simulink model "IEEE9_16b_Rockefeller_uderen"  (R2020a)
settings: Solver=ode8  StartTime=0.0  StopTime=5  MaxStep=1e-4  RelTol=1e-3
undefined symbols (not defined in the file or in its folder): k
libraries: powerlib x33, powerlib_meascontrol x27, simulink_extras x24, dspsigops x6, sps_avr x3
(part 2 of 2)

== system IEEE9_16b_Rockefeller_uderen/192 MW ==
  note: 18kV 192 MVA
  192 MVA : powerlib/Machines/Synchronous Machine pu Standard  PresetModel=No  MechanicalLoad=Mechanical power Pm  ShowDetailedParameters=on  RotorType=Salient-pole  Units=per unit standard parameters  MeasurementBus=off  NominalParameters="[192e6  18000   60 ]"  Reactances1=[ 31 32 33 34 35 36 37 ]  Reactances2=[ 1.305, 0.296, 0.252, 0.474, 0.243, 0.18 ]  dAxisTimeConstants=Short-circuit  qAxisTimeConstants=Open-circuit  TimeConstants1=[]  TimeConstants2=[]  TimeConstants3=[]  TimeConstants4=[]  TimeConstants5=[ 1.01, 0.053, 0.1 ]  TimeConstants6=[]  TimeConstants7=[]  TimeConstants8=[]  StatorResistance=2.8544e-3  Mechanical="[20 0  32]"  PolePairs=32  InitialConditions=[0 -73.0594 0.600015 0.600015 0.600015 0.71576 -119.284 120.716 1.18255]  SetSaturation=off  Saturation=[0.6404,0.7127,0.8441,0.9214,0.9956,1.082,1.19,1.316,1.457;0.7,0.7698,0.8872,0.9466,0.9969,1.046,1.1,1.151,1.201]  LoadFlowParameters=[1 500000000 0 0 0]  TsPowergui=0  TsBlock=-1  IterativeModel=Trapezoidal non iterative  IterativeDiscreteModel=Trapezoidal non iterative  BusType=PV  Pref=0.6*192e6  Qref=0  Qmin=-Inf  Qmax=Inf  PLF=0  QLF=0
      settings: AttributesFormatString=\n\n
  Pref3 : Constant  Value=0.6
  Reg_M1 : Subsystem
  A : PMIOPort  Side=Right
  B : PMIOPort  Port=2  Side=Right
  C : PMIOPort  Port=3  Side=Right
  wires:
  Reg_M1/1(Pm) -> 192 MVA/1
  192 MVA/1 -> Reg_M1/1(m)
  Reg_M1/2(Vf) -> 192 MVA/2
  Pref3/1 -> Reg_M1/2(Pref)
  connections:
  192 MVA/RConn1 -- A/RConn1
  192 MVA/RConn3 -- C/RConn1
  192 MVA/RConn2 -- B/RConn1

== system IEEE9_16b_Rockefeller_uderen/247.5 MW ==
  note: 16.5kV 247.5 MVA
  247.5 MVA : powerlib/Machines/Synchronous Machine pu Standard  PresetModel=No  MechanicalLoad=Mechanical power Pm  ShowDetailedParameters=on  RotorType=Salient-pole  Units=per unit standard parameters  MeasurementBus=off  NominalParameters="[247.5e6  16500   60 ]"  Reactances1=[ 31 32 33 34 35 36 37 ]  Reactances2=[ 1.305, 0.296, 0.252, 0.474, 0.243, 0.18 ]  dAxisTimeConstants=Short-circuit  qAxisTimeConstants=Open-circuit  TimeConstants1=[]  TimeConstants2=[]  TimeConstants3=[]  TimeConstants4=[]  TimeConstants5=[ 1.01, 0.053, 0.1 ]  TimeConstants6=[]  TimeConstants7=[]  TimeConstants8=[]  StatorResistance=2.8544e-3  Mechanical=[20 0 32]  PolePairs=32  InitialConditions=[0 -76.6925 0.514814 0.514814 0.514814 -5.74321 -125.743 114.257 1.19383]  SetSaturation=off  Saturation=[0.6404,0.7127,0.8441,0.9214,0.9956,1.082,1.19,1.316,1.457;0.7,0.7698,0.8872,0.9466,0.9969,1.046,1.1,1.151,1.201]  LoadFlowParameters=[1 500000000 0 0 0]  TsPowergui=0  TsBlock=-1  IterativeModel=Trapezoidal non iterative  IterativeDiscreteModel=Trapezoidal non iterative  BusType=swing  Pref=5e+008  Qref=0  Qmin=-Inf  Qmax=Inf  PLF=0  QLF=0
      settings: AttributesFormatString=\n\n
  Pref3 : Constant  Value=0.51223
  Reg_M1 : Subsystem
  A : PMIOPort  Side=Right
  B : PMIOPort  Port=2  Side=Right
  C : PMIOPort  Port=3  Side=Right
  wires:
  Reg_M1/1(Pm) -> 247.5 MVA/1
  Reg_M1/2(Vf) -> 247.5 MVA/2
  Pref3/1 -> Reg_M1/2(Pref)
  247.5 MVA/1 -> Reg_M1/1(m)
  connections:
  A/RConn1 -- 247.5 MVA/RConn1
  247.5 MVA/RConn2 -- B/RConn1
  247.5 MVA/RConn3 -- C/RConn1

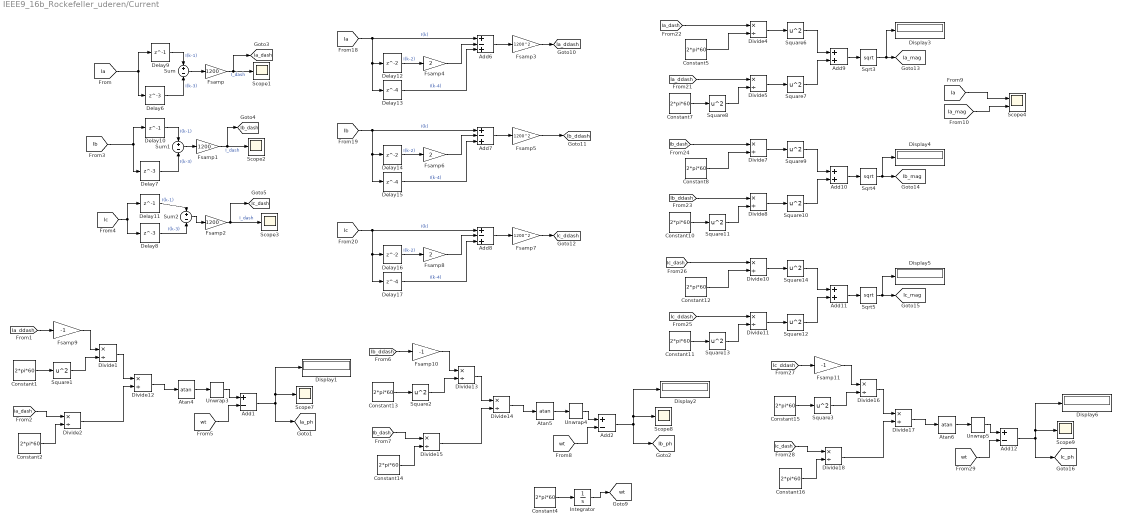
== system IEEE9_16b_Rockefeller_uderen/Current  ==
  Add1 : Sum  Inputs=+-
  Add10 : Sum
  Add11 : Sum
  Add12 : Sum  Inputs=+-
  Add2 : Sum  Inputs=+-
  Add6 : Sum  Inputs=+-+
  Add7 : Sum  Inputs=+-+
  Add8 : Sum  Inputs=+-+
  Add9 : Sum
  Atan4 : Trigonometry  Operator=atan
  Atan5 : Trigonometry  Operator=atan
  Atan6 : Trigonometry  Operator=atan
  Constant{1..2,4..5,7..8,10..16} (13 alike) : Constant  Value=2*pi*60
  Delay10 : Delay  DelayLength=1  SampleTime=1/1200
  Delay11 : Delay  DelayLength=1  SampleTime=1/1200
  Delay12 : Delay  SampleTime=1/1200
  Delay13 : Delay  DelayLength=4  SampleTime=1/1200
  Delay14 : Delay  SampleTime=1/1200
  Delay15 : Delay  DelayLength=4  SampleTime=1/1200
  Delay16 : Delay  SampleTime=1/1200
  Delay17 : Delay  DelayLength=4  SampleTime=1/1200
  Delay6 : Delay  DelayLength=3  SampleTime=1/1200
  Delay7 : Delay  DelayLength=3  SampleTime=1/1200
  Delay8 : Delay  DelayLength=3  SampleTime=1/1200
  Delay9 : Delay  DelayLength=1  SampleTime=1/1200
  Display{1..6} (6 alike) : Display
  Divide{1..2,4..5,7..8,10..18} (15 alike) : Product  Inputs=*/
  Fsamp : Gain  Gain=1200
  Fsamp1 : Gain  Gain=1200
  Fsamp10 : Gain  Gain=-1
  Fsamp11 : Gain  Gain=-1
  Fsamp2 : Gain  Gain=1200
  Fsamp3 : Gain  Gain=1200^2
  Fsamp4 : Gain  Gain=2
  Fsamp5 : Gain  Gain=1200^2
  Fsamp6 : Gain  Gain=2
  Fsamp7 : Gain  Gain=1200^2
  Fsamp8 : Gain  Gain=2
  Fsamp9 : Gain  Gain=-1
  Integrator : Integrator  WrappedStateUpperValue=2*pi  WrappedStateLowerValue=0
  Scope{1..3,7..9} (6 alike) : Scope
  Scope4 : Scope  NumInputPorts=2
  Sqrt3 : Sqrt  SaturateOnIntegerOverflow=on
  Sqrt4 : Sqrt  SaturateOnIntegerOverflow=on
  Sqrt5 : Sqrt  SaturateOnIntegerOverflow=on
  Square{1..3,6..14} (12 alike) : Math  Operator=square  SaturateOnIntegerOverflow=on
  Sum : Sum  Inputs=+-
  Sum1 : Sum  Inputs=+-
  Sum2 : Sum  Inputs=+-
  Unwrap3 : dspsigops/Unwrap  tol=-2*pi  InputProcessing=Columns as channels (frame based)  running=off
  Unwrap4 : dspsigops/Unwrap  tol=-2*pi  InputProcessing=Columns as channels (frame based)  running=off
  Unwrap5 : dspsigops/Unwrap  tol=-2*pi  InputProcessing=Columns as channels (frame based)  running=off
  tag scope: Ia_dash=global, Ia_ddash=global, Ia_mag=global, Ia_ph=global, Ib_dash=global, Ib_ddash=global, Ib_mag=global, Ib_ph=global, Ic_dash=global, Ic_ddash=global, Ic_mag=global, Ic_ph=global, wt=global
  wires:
  Delay6/1 -> Sum/2  "I(k-3)"
  [Ia] -> Delay6/1, Delay9/1
  Fsamp2/1 -> [Ic_dash], Scope3/1  "I_dash"
  Fsamp/1 -> [Ia_dash], Scope1/1  "I_dash"
  Sum1/1 -> Fsamp1/1
  Sum/1 -> Fsamp/1
  Constant4/1 -> Integrator/1
  Integrator/1 -> [wt]
  Delay9/1 -> Sum/1  "I(k-1)"
  Delay10/1 -> Sum1/1  "I(k-1)"
  [Ib] -> Delay7/1, Delay10/1
  Delay7/1 -> Sum1/2  "I(k-3)"
  Fsamp1/1 -> [Ib_dash], Scope2/1  "I_dash"
  Delay11/1 -> Sum2/1  "I(k-1)"
  [Ic] -> Delay8/1, Delay11/1
  Delay8/1 -> Sum2/2  "I(k-3)"
  Sum2/1 -> Fsamp2/1
  Delay12/1 -> Fsamp4/1  "I(k-2)"
  [Ia] -> Delay13/1, Delay12/1, Add6/1  "I(k)"
  Fsamp4/1 -> Add6/2
  Delay13/1 -> Add6/3  "I(k-4)"
  Add6/1 -> Fsamp3/1
  Fsamp3/1 -> [Ia_ddash]
  Fsamp5/1 -> [Ib_ddash]
  Add7/1 -> Fsamp5/1
  Delay15/1 -> Add7/3  "I(k-4)"
  Fsamp6/1 -> Add7/2
  [Ib] -> Add7/1, Delay14/1, Delay15/1  "I(k)"
  Delay14/1 -> Fsamp6/1  "I(k-2)"
  Delay16/1 -> Fsamp8/1  "I(k-2)"
  [Ic] -> Delay17/1, Delay16/1, Add8/1  "I(k)"
  Fsamp8/1 -> Add8/2
  Delay17/1 -> Add8/3  "I(k-4)"
  Add8/1 -> Fsamp7/1
  Fsamp7/1 -> [Ic_ddash]
  Constant5/1 -> Divide4/2
  Divide4/1 -> Square6/1
  [Ia_ddash] -> Divide5/1
  Divide5/1 -> Square7/1
  Constant7/1 -> Square8/1
  Square8/1 -> Divide5/2
  Square6/1 -> Add9/1
  Square7/1 -> Add9/2
  Add9/1 -> Sqrt3/1
  Sqrt3/1 -> Display3/1, [Ia_mag]
  Sqrt4/1 -> Display4/1, [Ib_mag]
  Add10/1 -> Sqrt4/1
  Square10/1 -> Add10/2
  Square9/1 -> Add10/1
  Square11/1 -> Divide8/2
  Constant10/1 -> Square11/1
  Divide8/1 -> Square10/1
  [Ib_ddash] -> Divide8/1
  Divide7/1 -> Square9/1
  Constant8/1 -> Divide7/2
  Constant12/1 -> Divide10/2
  Divide10/1 -> Square14/1
  [Ic_ddash] -> Divide11/1
  Divide11/1 -> Square12/1
  Constant11/1 -> Square13/1
  Square13/1 -> Divide11/2
  Square14/1 -> Add11/1
  Square12/1 -> Add11/2
  Add11/1 -> Sqrt5/1
  Sqrt5/1 -> Display5/1, [Ic_mag]
  [Ia_dash] -> Divide4/1
  [Ib_dash] -> Divide7/1
  [Ic_dash] -> Divide10/1
  [Ia_ddash] -> Fsamp9/1
  Constant1/1 -> Square1/1
  Fsamp9/1 -> Divide1/1
  Square1/1 -> Divide1/2
  [Ia_dash] -> Divide2/1
  Constant2/1 -> Divide2/2
  Divide1/1 -> Divide12/1
  Divide2/1 -> Divide12/2
  Divide12/1 -> Atan4/1
  Atan4/1 -> Unwrap3/1
  Unwrap3/1 -> Add1/1
  [wt] -> Add1/2
  Add1/1 -> Display1/1, Scope7/1, [Ia_ph]
  Add2/1 -> [Ib_ph], Scope8/1, Display2/1
  [wt] -> Add2/2
  Unwrap4/1 -> Add2/1
  Atan5/1 -> Unwrap4/1
  Divide14/1 -> Atan5/1
  Divide15/1 -> Divide14/2
  Divide13/1 -> Divide14/1
  Constant14/1 -> Divide15/2
  [Ib_dash] -> Divide15/1
  Square2/1 -> Divide13/2
  Fsamp10/1 -> Divide13/1
  Constant13/1 -> Square2/1
  [Ib_ddash] -> Fsamp10/1
  [Ic_ddash] -> Fsamp11/1
  Constant15/1 -> Square3/1
  Fsamp11/1 -> Divide16/1
  Square3/1 -> Divide16/2
  [Ic_dash] -> Divide18/1
  Constant16/1 -> Divide18/2
  Divide16/1 -> Divide17/1
  Divide18/1 -> Divide17/2
  Divide17/1 -> Atan6/1
  Atan6/1 -> Unwrap5/1
  Unwrap5/1 -> Add12/1
  [wt] -> Add12/2
  Add12/1 -> Display6/1, Scope9/1, [Ic_ph]
  [Ia] -> Scope4/1
  [Ia_mag] -> Scope4/2

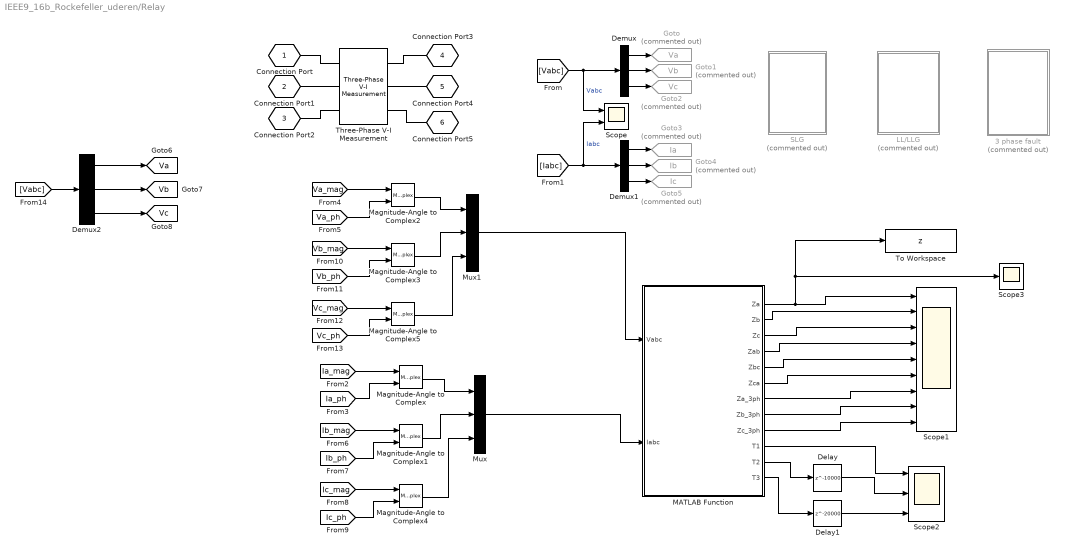
== system IEEE9_16b_Rockefeller_uderen/Relay ==
  3 phase fault : Subsystem  Commented=on
  Delay : Delay  DelayLength=10000  SampleTime=50e-6
  Delay1 : Delay  DelayLength=20000  SampleTime=50e-6
  Demux : Demux  Outputs=3
  Demux1 : Demux  Outputs=3
  Demux2 : Demux  Outputs=3
  Goto : Goto  Commented=on  GotoTag=Va  TagVisibility=global
  Goto1 : Goto  Commented=on  GotoTag=Vb  TagVisibility=global
  Goto2 : Goto  Commented=on  GotoTag=Vc  TagVisibility=global
  Goto3 : Goto  Commented=on  GotoTag=Ia  TagVisibility=global
  Goto4 : Goto  Commented=on  GotoTag=Ib  TagVisibility=global
  Goto5 : Goto  Commented=on  GotoTag=Ic  TagVisibility=global
  LL/LLG : Subsystem  Commented=on
  MATLAB Function : MATLAB Function  TreatAsAtomicUnit=on
  Magnitude-Angle to Complex{,1..5} (6 alike) : MagnitudeAngleToComplex
  Mux : Mux  Inputs=3
  Mux1 : Mux  Inputs=3
  SLG : Subsystem  Commented=on
  Scope : Scope  NumInputPorts=2
  Scope1 : Scope  NumInputPorts=9
  Scope2 : Scope  NumInputPorts=3
  Scope3 : Scope
  Three-Phase V-I Measurement : powerlib/Measurements/Three-Phase V-I Measurement  VoltageMeasurement=phase-to-ground  SetLabelV=on  LabelV=Vabc  Vpu=off  VpuLL=off  CurrentMeasurement=yes  SetLabelI=on  LabelI=Iabc  Ipu=off  Pbase=100e6  Vbase=500e3  OutputType=Complex  PhasorSimulation=off  PSBequivalent=0
  To Workspace : ToWorkspace  VariableName=z  SampleTime=-1
  Connection Port : PMIOPort  Tag=PMCPort  Side=Left
  Connection Port1 : PMIOPort  Tag=PMCPort  Port=2  Side=Left
  Connection Port2 : PMIOPort  Tag=PMCPort  Port=3  Side=Left
  Connection Port3 : PMIOPort  Tag=PMCPort  Port=4  Side=Right
  Connection Port4 : PMIOPort  Tag=PMCPort  Port=5  Side=Right
  Connection Port5 : PMIOPort  Tag=PMCPort  Port=6  Side=Right
  tag scope: Va=global, Vb=global, Vc=global
  wires:
  Demux1/3 -> Goto5/1
  Demux1/1 -> Goto3/1
  Demux/3 -> Goto2/1
  Demux/1 -> Goto/1
  Demux/2 -> Goto1/1
  [Iabc] -> Scope/2, Demux1/1  "Iabc"
  [Vabc] -> Scope/1, Demux/1  "Vabc"
  Demux1/2 -> Goto4/1
  MATLAB Function/1(Za) -> Scope3/1, To Workspace/1, Scope1/1
  MATLAB Function/2(Zb) -> Scope1/2
  MATLAB Function/3(Zc) -> Scope1/3
  MATLAB Function/4(Zab) -> Scope1/4
  MATLAB Function/5(Zbc) -> Scope1/5
  MATLAB Function/6(Zca) -> Scope1/6
  MATLAB Function/10(T1) -> Scope2/1
  Mux/1 -> MATLAB Function/2(Iabc)
  MATLAB Function/11(T2) -> Delay/1
  MATLAB Function/12(T3) -> Delay1/1
  Delay/1 -> Scope2/2
  Delay1/1 -> Scope2/3
  MATLAB Function/7(Za_3ph) -> Scope1/7
  MATLAB Function/8(Zb_3ph) -> Scope1/8
  MATLAB Function/9(Zc_3ph) -> Scope1/9
  [Ia_mag] -> Magnitude-Angle to Complex/1
  [Ia_ph] -> Magnitude-Angle to Complex/2
  [Ib_ph] -> Magnitude-Angle to Complex1/2
  [Ib_mag] -> Magnitude-Angle to Complex1/1
  [Ic_mag] -> Magnitude-Angle to Complex4/1
  [Ic_ph] -> Magnitude-Angle to Complex4/2
  Magnitude-Angle to Complex/1 -> Mux/1
  Magnitude-Angle to Complex1/1 -> Mux/2
  Magnitude-Angle to Complex4/1 -> Mux/3
  Magnitude-Angle to Complex5/1 -> Mux1/3
  Magnitude-Angle to Complex3/1 -> Mux1/2
  Magnitude-Angle to Complex2/1 -> Mux1/1
  [Vc_ph] -> Magnitude-Angle to Complex5/2
  [Vc_mag] -> Magnitude-Angle to Complex5/1
  [Vb_mag] -> Magnitude-Angle to Complex3/1
  [Vb_ph] -> Magnitude-Angle to Complex3/2
  [Va_ph] -> Magnitude-Angle to Complex2/2
  [Va_mag] -> Magnitude-Angle to Complex2/1
  Mux1/1 -> MATLAB Function/1(Vabc)
  [Vabc] -> Demux2/1
  Demux2/1 -> [Va]
  Demux2/2 -> [Vb]
  Demux2/3 -> [Vc]
  connections:
  Connection Port/RConn1 -- Three-Phase V-I Measurement/LConn1
  Connection Port1/RConn1 -- Three-Phase V-I Measurement/LConn2
  Connection Port2/RConn1 -- Three-Phase V-I Measurement/LConn3
  Connection Port3/RConn1 -- Three-Phase V-I Measurement/RConn1
  Connection Port4/RConn1 -- Three-Phase V-I Measurement/RConn2
  Connection Port5/RConn1 -- Three-Phase V-I Measurement/RConn3

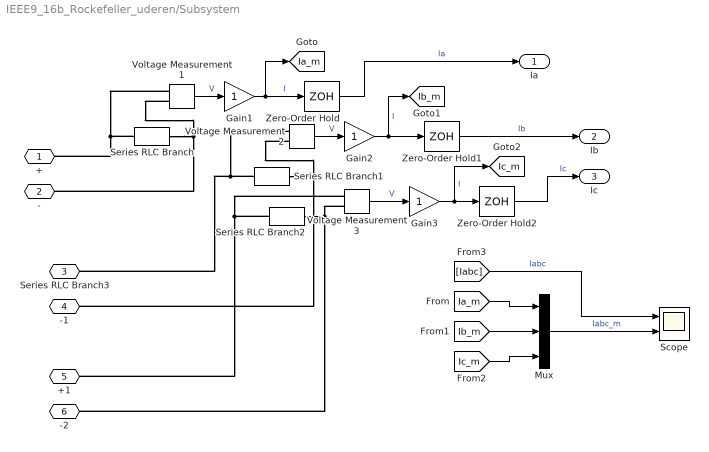
== system IEEE9_16b_Rockefeller_uderen/Subsystem ==
  Gain1 : Gain
  Gain2 : Gain
  Gain3 : Gain
  Mux : Mux  Inputs=3
  Scope : Scope  NumInputPorts=2
  Series RLC Branch : powerlib/Elements/Series RLC Branch  LConnTagsString=__new0  RConnTagsString=__new0  BranchType=RL  Resistance=0.11727  Inductance=2.634e-3  SetiL0=off  InitialCurrent=0  Capacitance=1e-6  Setx0=off  InitialVoltage=0  Measurements=None
  Series RLC Branch1 : powerlib/Elements/Series RLC Branch  LConnTagsString=__new0  RConnTagsString=__new0  BranchType=RL  Resistance=0.11727  Inductance=2.634e-3  SetiL0=off  InitialCurrent=0  Capacitance=1e-6  Setx0=off  InitialVoltage=0  Measurements=None
  Series RLC Branch2 : powerlib/Elements/Series RLC Branch  LConnTagsString=__new0  RConnTagsString=__new0  BranchType=RL  Resistance=0.11727  Inductance=2.634e-3  SetiL0=off  InitialCurrent=0  Capacitance=1e-6  Setx0=off  InitialVoltage=0  Measurements=None
  Voltage Measurement1 : powerlib/Measurements/Voltage Measurement  PhasorSimulation=off  OutputType=Complex  PSBequivalent=0
  Voltage Measurement2 : powerlib/Measurements/Voltage Measurement  PhasorSimulation=off  OutputType=Complex  PSBequivalent=0
  Voltage Measurement3 : powerlib/Measurements/Voltage Measurement  PhasorSimulation=off  OutputType=Complex  PSBequivalent=0
  Zero-Order Hold : ZeroOrderHold  SampleTime=1/1200
  Zero-Order Hold1 : ZeroOrderHold  SampleTime=1/1200
  Zero-Order Hold2 : ZeroOrderHold  SampleTime=1/1200
  + : PMIOPort  Side=Left
  - : PMIOPort  Port=2  Side=Left
  Series RLC Branch3 : PMIOPort  Port=3  Side=Left
  -1 : PMIOPort  Port=4  Side=Left
  +1 : PMIOPort  Port=5  Side=Left
  -2 : PMIOPort  Port=6  Side=Left
  Ia : Outport
  Ib : Outport  Port=2
  Ic : Outport  Port=3
  tag scope: Ia_m=global, Ib_m=global, Ic_m=global
  wires:
  Voltage Measurement1/1 -> Gain1/1  "V"
  Gain1/1 -> [Ia_m], Zero-Order Hold/1  "I"
  Voltage Measurement2/1 -> Gain2/1  "V"
  Gain2/1 -> [Ib_m], Zero-Order Hold1/1  "I"
  Zero-Order Hold1/1 -> Ib/1  "Ib"
  Voltage Measurement3/1 -> Gain3/1  "V"
  Gain3/1 -> [Ic_m], Zero-Order Hold2/1  "I"
  Zero-Order Hold/1 -> Ia/1  "Ia"
  Zero-Order Hold2/1 -> Ic/1  "Ic"
  [Ib_m] -> Mux/2
  [Ic_m] -> Mux/3
  [Ia_m] -> Mux/1
  Mux/1 -> Scope/2  "Iabc_m"
  [Iabc] -> Scope/1  "Iabc"
  connections:
  Series RLC Branch2/LConn1 -- +1/RConn1 -- Voltage Measurement3/LConn1
  Series RLC Branch/LConn1 -- +/RConn1 -- Voltage Measurement1/LConn1
  Series RLC Branch2/RConn1 -- -2/RConn1 -- Voltage Measurement3/LConn2
  Series RLC Branch1/RConn1 -- -1/RConn1 -- Voltage Measurement2/LConn2
  Voltage Measurement2/LConn1 -- Series RLC Branch3/RConn1 -- Series RLC Branch1/LConn1
  Series RLC Branch/RConn1 -- -/RConn1 -- Voltage Measurement1/LConn2

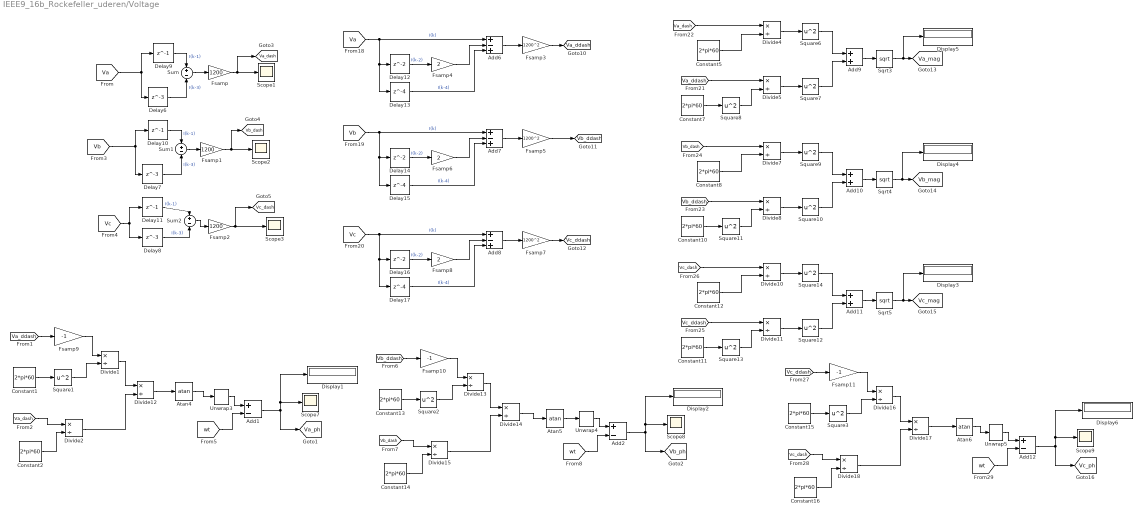
== system IEEE9_16b_Rockefeller_uderen/Voltage ==
  Add1 : Sum  Inputs=+-
  Add10 : Sum
  Add11 : Sum
  Add12 : Sum  Inputs=+-
  Add2 : Sum  Inputs=+-
  Add6 : Sum  Inputs=+-+
  Add7 : Sum  Inputs=+-+
  Add8 : Sum  Inputs=+-+
  Add9 : Sum
  Atan4 : Trigonometry  Operator=atan
  Atan5 : Trigonometry  Operator=atan
  Atan6 : Trigonometry  Operator=atan
  Constant{1..2,5,7..8,10..16} (12 alike) : Constant  Value=2*pi*60
  Delay10 : Delay  DelayLength=1  SampleTime=1/1200
  Delay11 : Delay  DelayLength=1  SampleTime=1/1200
  Delay12 : Delay  SampleTime=1/1200
  Delay13 : Delay  DelayLength=4  SampleTime=1/1200
  Delay14 : Delay  SampleTime=1/1200
  Delay15 : Delay  DelayLength=4  SampleTime=1/1200
  Delay16 : Delay  SampleTime=1/1200
  Delay17 : Delay  DelayLength=4  SampleTime=1/1200
  Delay6 : Delay  DelayLength=3  SampleTime=1/1200
  Delay7 : Delay  DelayLength=3  SampleTime=1/1200
  Delay8 : Delay  DelayLength=3  SampleTime=1/1200
  Delay9 : Delay  DelayLength=1  SampleTime=1/1200
  Display{1..6} (6 alike) : Display
  Divide{1..2,4..5,7..8,10..18} (15 alike) : Product  Inputs=*/
  Fsamp : Gain  Gain=1200
  Fsamp1 : Gain  Gain=1200
  Fsamp10 : Gain  Gain=-1
  Fsamp11 : Gain  Gain=-1
  Fsamp2 : Gain  Gain=1200
  Fsamp3 : Gain  Gain=1200^2
  Fsamp4 : Gain  Gain=2
  Fsamp5 : Gain  Gain=1200^2
  Fsamp6 : Gain  Gain=2
  Fsamp7 : Gain  Gain=1200^2
  Fsamp8 : Gain  Gain=2
  Fsamp9 : Gain  Gain=-1
  Scope{1..3,7..9} (6 alike) : Scope
  Sqrt3 : Sqrt  SaturateOnIntegerOverflow=on
  Sqrt4 : Sqrt  SaturateOnIntegerOverflow=on
  Sqrt5 : Sqrt  SaturateOnIntegerOverflow=on
  Square{1..3,6..14} (12 alike) : Math  Operator=square  SaturateOnIntegerOverflow=on
  Sum : Sum  Inputs=+-
  Sum1 : Sum  Inputs=+-
  Sum2 : Sum  Inputs=+-
  Unwrap3 : dspsigops/Unwrap  tol=-2*pi  InputProcessing=Columns as channels (frame based)  running=off
  Unwrap4 : dspsigops/Unwrap  tol=-2*pi  InputProcessing=Columns as channels (frame based)  running=off
  Unwrap5 : dspsigops/Unwrap  tol=-2*pi  InputProcessing=Columns as channels (frame based)  running=off
  tag scope: Va_dash=global, Va_ddash=global, Va_mag=global, Va_ph=global, Vb_dash=global, Vb_ddash=global, Vb_mag=global, Vb_ph=global, Vc_dash=global, Vc_ddash=global, Vc_mag=global, Vc_ph=global
  wires:
  Add12/1 -> [Vc_ph], Scope9/1, Display6/1
  [wt] -> Add12/2
  Unwrap5/1 -> Add12/1
  Atan6/1 -> Unwrap5/1
  Divide17/1 -> Atan6/1
  Divide18/1 -> Divide17/2
  Divide16/1 -> Divide17/1
  Constant16/1 -> Divide18/2
  [Vc_dash] -> Divide18/1
  Square3/1 -> Divide16/2
  Fsamp11/1 -> Divide16/1
  Constant15/1 -> Square3/1
  [Vc_ddash] -> Fsamp11/1
  [Vb_ddash] -> Fsamp10/1
  Constant13/1 -> Square2/1
  Fsamp10/1 -> Divide13/1
  Square2/1 -> Divide13/2
  [Vb_dash] -> Divide15/1
  Constant14/1 -> Divide15/2
  Divide13/1 -> Divide14/1
  Divide15/1 -> Divide14/2
  Divide14/1 -> Atan5/1
  Atan5/1 -> Unwrap4/1
  Unwrap4/1 -> Add2/1
  [wt] -> Add2/2
  Add2/1 -> Display2/1, Scope8/1, [Vb_ph]
  Add1/1 -> [Va_ph], Scope7/1, Display1/1
  [wt] -> Add1/2
  Unwrap3/1 -> Add1/1
  Atan4/1 -> Unwrap3/1
  Divide12/1 -> Atan4/1
  Divide2/1 -> Divide12/2
  Divide1/1 -> Divide12/1
  Constant2/1 -> Divide2/2
  [Va_dash] -> Divide2/1
  Square1/1 -> Divide1/2
  Fsamp9/1 -> Divide1/1
  Constant1/1 -> Square1/1
  [Va_ddash] -> Fsamp9/1
  [Vc_dash] -> Divide10/1
  [Vb_dash] -> Divide7/1
  [Va_dash] -> Divide4/1
  Sqrt5/1 -> Display3/1, [Vc_mag]
  Add11/1 -> Sqrt5/1
  Square12/1 -> Add11/2
  Square14/1 -> Add11/1
  Square13/1 -> Divide11/2
  Constant11/1 -> Square13/1
  Divide11/1 -> Square12/1
  [Vc_ddash] -> Divide11/1
  Divide10/1 -> Square14/1
  Constant12/1 -> Divide10/2
  Constant8/1 -> Divide7/2
  Divide7/1 -> Square9/1
  [Vb_ddash] -> Divide8/1
  Divide8/1 -> Square10/1
  Constant10/1 -> Square11/1
  Square11/1 -> Divide8/2
  Square9/1 -> Add10/1
  Square10/1 -> Add10/2
  Add10/1 -> Sqrt4/1
  Sqrt4/1 -> Display4/1, [Vb_mag]
  Sqrt3/1 -> Display5/1, [Va_mag]
  Add9/1 -> Sqrt3/1
  Square7/1 -> Add9/2
  Square6/1 -> Add9/1
  Square8/1 -> Divide5/2
  Constant7/1 -> Square8/1
  Divide5/1 -> Square7/1
  [Va_ddash] -> Divide5/1
  Divide4/1 -> Square6/1
  Constant5/1 -> Divide4/2
  Fsamp7/1 -> [Vc_ddash]
  Add8/1 -> Fsamp7/1
  Delay17/1 -> Add8/3  "I(k-4)"
  Fsamp8/1 -> Add8/2
  [Vc] -> Add8/1, Delay16/1, Delay17/1  "I(k)"
  Delay16/1 -> Fsamp8/1  "I(k-2)"
  Delay14/1 -> Fsamp6/1  "I(k-2)"
  [Vb] -> Delay15/1, Delay14/1, Add7/1  "I(k)"
  Fsamp6/1 -> Add7/2
  Delay15/1 -> Add7/3  "I(k-4)"
  Add7/1 -> Fsamp5/1
  Fsamp5/1 -> [Vb_ddash]
  Fsamp3/1 -> [Va_ddash]
  Add6/1 -> Fsamp3/1
  Delay13/1 -> Add6/3  "I(k-4)"
  Fsamp4/1 -> Add6/2
  [Va] -> Add6/1, Delay12/1, Delay13/1  "I(k)"
  Delay12/1 -> Fsamp4/1  "I(k-2)"
  Sum2/1 -> Fsamp2/1
  Delay8/1 -> Sum2/2  "I(k-3)"
  [Vc] -> Delay11/1, Delay8/1
  Delay11/1 -> Sum2/1  "I(k-1)"
  Fsamp1/1 -> Scope2/1, [Vb_dash]
  Delay7/1 -> Sum1/2  "I(k-3)"
  [Vb] -> Delay10/1, Delay7/1
  Delay10/1 -> Sum1/1  "I(k-1)"
  Delay9/1 -> Sum/1  "I(k-1)"
  Sum/1 -> Fsamp/1
  Sum1/1 -> Fsamp1/1
  Fsamp/1 -> Scope1/1, [Va_dash]
  Fsamp2/1 -> Scope3/1, [Vc_dash]
  [Va] -> Delay9/1, Delay6/1
  Delay6/1 -> Sum/2  "I(k-3)"

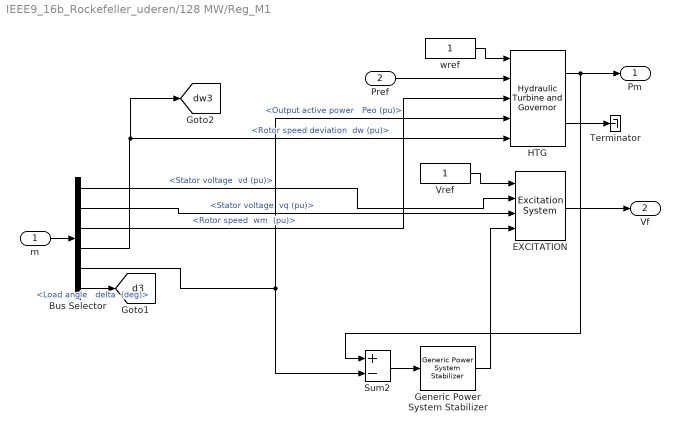
== system IEEE9_16b_Rockefeller_uderen/128 MW/Reg_M1 ==
  m : Inport
  Pref : Inport  Port=2
  Bus Selector : BusSelector  OutputSignals="dq0 components.Stator voltage  vd (pu),dq0 components.Stator voltage  vq (pu),Mechanical.Rotor speed  wm  (pu),Mechanical.Rotor speed deviation  dw (pu),Output active power   Peo (pu),Load angle   delta  (deg)"
  EXCITATION : sps_avr/Excitation System  tr=20e-3  reg=[ 200, 0.001 ]  exc=[ 1, 0 ]  tgr=[ 0, 0 ]  damp=[ 0.001, 0.1 ]  sat=[ 0, 0 ]  lim="[ 0,  7, 0 ]"  v0=[1 1.1034]
      settings: SourceProductBaseCode=PS
  Generic Power System Stabilizer : powerlib/Machines/Generic Power System Stabilizer  Tsensor=15e-3  K=2.5  Twashout=1  Tleadlag1="[0.06  1]"  Tleadlag2="[0  0]"  VSlimits=[-0.15 0.15]  Vinit=0  Plot_On=off  MagdB_On=on  FreqRange=logspace(-2,2,500)
      settings: SourceProductBaseCode=PS
  HTG : powerlib/Machines/Hydraulic Turbine and Governor  sm="[ 10/3  0.07 ]"  gate="[  0.01  0.97518  -0.1  0.1 ]"  reg="[  0.05  1.163  0.105  0  0.01  ]"  hyd="[  0  2.67  ]"  dref=0  po=0.60104
      settings: SourceProductBaseCode=PS
  Sum2 : Sum  Inputs=+-  InputSameDT=on  SaturateOnIntegerOverflow=on  OutDataTypeStr=Inherit: Same as first input
  Terminator : Terminator
  Vref : Constant
  wref : Constant
  Pm : Outport  InitialOutput=0
  Vf : Outport  Port=2  InitialOutput=0
  tag scope: d3=global, dw3=global
  wires:
  HTG/2 -> Terminator/1
  Vref/1 -> EXCITATION/1
  m/1 -> Bus Selector/1
  Bus Selector/4 -> [dw3], HTG/5  "<Rotor speed deviation  dw (pu)>"
  Bus Selector/5 -> HTG/4, Sum2/2  "<Output active power   Peo (pu)>"
  Bus Selector/3 -> HTG/3  "<Rotor speed  wm  (pu)>"
  Pref/1 -> HTG/2
  wref/1 -> HTG/1
  HTG/1 -> Pm/1, Sum2/1
  Bus Selector/2 -> EXCITATION/3  "<Stator voltage  vq (pu)>"
  EXCITATION/1 -> Vf/1
  Bus Selector/1 -> EXCITATION/2  "<Stator voltage  vd (pu)>"
  Generic Power System Stabilizer/1 -> EXCITATION/4
  Sum2/1 -> Generic Power System Stabilizer/1
  Bus Selector/6 -> [d3]  "<Load angle   delta  (deg)>"

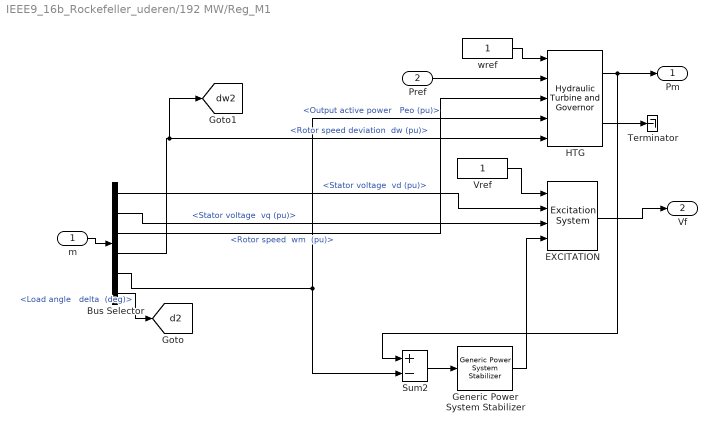
== system IEEE9_16b_Rockefeller_uderen/192 MW/Reg_M1 ==
  m : Inport
  Pref : Inport  Port=2
  Bus Selector : BusSelector  OutputSignals="dq0 components.Stator voltage  vd (pu),dq0 components.Stator voltage  vq (pu),Mechanical.Rotor speed  wm  (pu),Mechanical.Rotor speed deviation  dw (pu),Output active power   Peo (pu),Load angle   delta  (deg)"
  EXCITATION : sps_avr/Excitation System  tr=20e-3  reg=[ 200, 0.001 ]  exc=[ 1, 0 ]  tgr=[ 0, 0 ]  damp=[ 0.001, 0.1 ]  sat=[ 0, 0 ]  lim="[ 0,  7, 0 ]"  v0=[1 1.1826]
      settings: SourceProductBaseCode=PS
  Generic Power System Stabilizer : powerlib/Machines/Generic Power System Stabilizer  Tsensor=15e-3  K=2.5  Twashout=1  Tleadlag1="[0.06  1]"  Tleadlag2="[0  0]"  VSlimits=[-0.15 0.15]  Vinit=0  Plot_On=off  MagdB_On=on  FreqRange=logspace(-2,2,500)
      settings: SourceProductBaseCode=PS
  HTG : powerlib/Machines/Hydraulic Turbine and Governor  sm="[ 10/3  0.07 ]"  gate="[  0.01  0.97518  -0.1  0.1 ]"  reg="[  0.05  1.163  0.105  0  0.01  ]"  hyd="[  0  2.67  ]"  dref=0  po=0.60103
      settings: SourceProductBaseCode=PS
  Sum2 : Sum  Inputs=+-  InputSameDT=on  SaturateOnIntegerOverflow=on  OutDataTypeStr=Inherit: Same as first input
  Terminator : Terminator
  Vref : Constant
  wref : Constant
  Pm : Outport  InitialOutput=0
  Vf : Outport  Port=2  InitialOutput=0
  tag scope: d2=global, dw2=global
  wires:
  HTG/2 -> Terminator/1
  Vref/1 -> EXCITATION/1
  m/1 -> Bus Selector/1
  Bus Selector/4 -> [dw2], HTG/5  "<Rotor speed deviation  dw (pu)>"
  Bus Selector/5 -> HTG/4, Sum2/2  "<Output active power   Peo (pu)>"
  Bus Selector/3 -> HTG/3  "<Rotor speed  wm  (pu)>"
  Pref/1 -> HTG/2
  wref/1 -> HTG/1
  HTG/1 -> Pm/1, Sum2/1
  Bus Selector/2 -> EXCITATION/3  "<Stator voltage  vq (pu)>"
  EXCITATION/1 -> Vf/1
  Bus Selector/1 -> EXCITATION/2  "<Stator voltage  vd (pu)>"
  Generic Power System Stabilizer/1 -> EXCITATION/4
  Sum2/1 -> Generic Power System Stabilizer/1
  Bus Selector/6 -> [d2]  "<Load angle   delta  (deg)>"

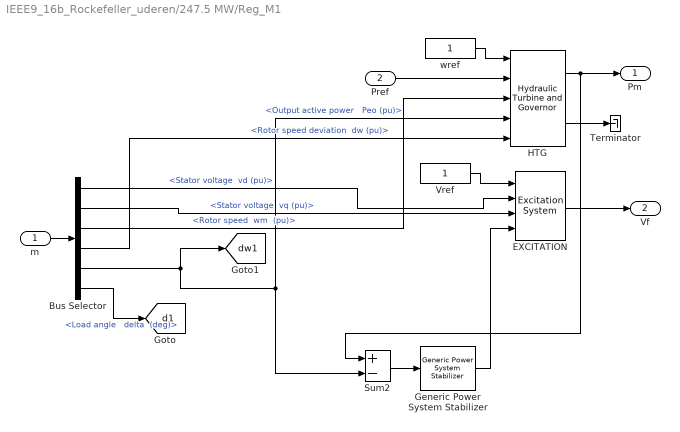
== system IEEE9_16b_Rockefeller_uderen/247.5 MW/Reg_M1 ==
  m : Inport
  Pref : Inport  Port=2
  Bus Selector : BusSelector  OutputSignals="dq0 components.Stator voltage  vd (pu),dq0 components.Stator voltage  vq (pu),Mechanical.Rotor speed  wm  (pu),Mechanical.Rotor speed deviation  dw (pu),Output active power   Peo (pu),Load angle   delta  (deg)"
  EXCITATION : sps_avr/Excitation System  tr=20e-3  reg=[ 200, 0.001 ]  exc=[ 1, 0 ]  tgr=[ 0, 0 ]  damp=[ 0.001, 0.1 ]  sat=[ 0, 0 ]  lim="[ 0,  7, 0 ]"  v0=[1 1.1938]
      settings: SourceProductBaseCode=PS
  Generic Power System Stabilizer : powerlib/Machines/Generic Power System Stabilizer  Tsensor=15e-3  K=2.5  Twashout=1  Tleadlag1="[0.06  1]"  Tleadlag2="[0  0]"  VSlimits=[-0.15 0.15]  Vinit=0  Plot_On=off  MagdB_On=on  FreqRange=logspace(-2,2,500)
      settings: SourceProductBaseCode=PS
  HTG : powerlib/Machines/Hydraulic Turbine and Governor  sm="[ 10/3  0.07 ]"  gate="[  0.01  0.97518  -0.1  0.1 ]"  reg="[  0.05  1.163  0.105  0  0.01  ]"  hyd="[  0  2.67  ]"  dref=0  po=0.51299
      settings: SourceProductBaseCode=PS
  Sum2 : Sum  Inputs=+-  InputSameDT=on  SaturateOnIntegerOverflow=on  OutDataTypeStr=Inherit: Same as first input
  Terminator : Terminator
  Vref : Constant
  wref : Constant
  Pm : Outport  InitialOutput=0
  Vf : Outport  Port=2  InitialOutput=0
  tag scope: d1=global, dw1=global
  wires:
  HTG/2 -> Terminator/1
  Vref/1 -> EXCITATION/1
  m/1 -> Bus Selector/1
  Bus Selector/4 -> HTG/5  "<Rotor speed deviation  dw (pu)>"
  Bus Selector/5 -> [dw1], HTG/4, Sum2/2  "<Output active power   Peo (pu)>"
  Bus Selector/3 -> HTG/3  "<Rotor speed  wm  (pu)>"
  Pref/1 -> HTG/2
  wref/1 -> HTG/1
  HTG/1 -> Pm/1, Sum2/1
  Bus Selector/2 -> EXCITATION/3  "<Stator voltage  vq (pu)>"
  EXCITATION/1 -> Vf/1
  Bus Selector/1 -> EXCITATION/2  "<Stator voltage  vd (pu)>"
  Generic Power System Stabilizer/1 -> EXCITATION/4
  Sum2/1 -> Generic Power System Stabilizer/1
  Bus Selector/6 -> [d1]  "<Load angle   delta  (deg)>"

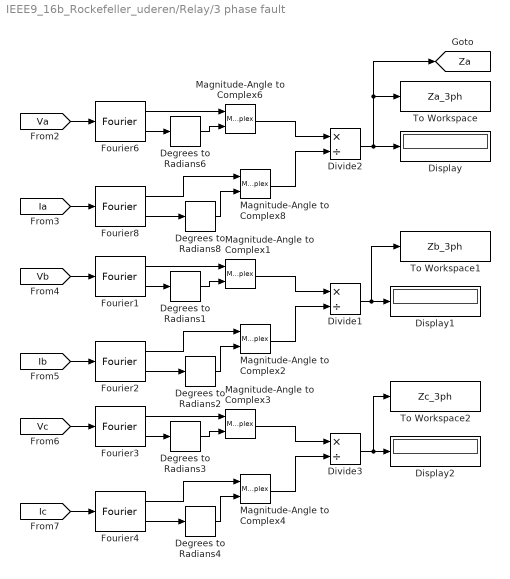
== system IEEE9_16b_Rockefeller_uderen/Relay/3 phase fault ==
  Degrees to Radians{1..4,6,8} (6 alike) : simulink_extras/Transformations/Degrees to Radians
  Display : Display
  Display1 : Display
  Display2 : Display
  Divide1 : Product  Inputs=*/
  Divide2 : Product  Inputs=*/
  Divide3 : Product  Inputs=*/
  Fourier{1..4,6,8} (6 alike) : powerlib_meascontrol/Measurements/Fourier  Freq=60  n=1  InInit=[0, 0]  Ts=0
  Magnitude-Angle to Complex{1..4,6,8} (6 alike) : MagnitudeAngleToComplex
  To Workspace : ToWorkspace  VariableName=Za_3ph  SaveFormat=Timeseries  SampleTime=-1
  To Workspace1 : ToWorkspace  VariableName=Zb_3ph  SaveFormat=Timeseries  SampleTime=-1
  To Workspace2 : ToWorkspace  VariableName=Zc_3ph  SaveFormat=Timeseries  SampleTime=-1
  tag scope: Za=global
  wires:
  Divide1/1 -> To Workspace1/1, Display1/1
  [Ia] -> Fourier8/1
  [Ib] -> Fourier2/1
  Degrees to Radians4/1 -> Magnitude-Angle to Complex4/2
  Magnitude-Angle to Complex3/1 -> Divide3/1
  Fourier4/2 -> Degrees to Radians4/1
  Degrees to Radians8/1 -> Magnitude-Angle to Complex8/2
  Fourier6/2 -> Degrees to Radians6/1
  Magnitude-Angle to Complex6/1 -> Divide2/1
  Magnitude-Angle to Complex8/1 -> Divide2/2
  Degrees to Radians2/1 -> Magnitude-Angle to Complex2/2
  Fourier8/2 -> Degrees to Radians8/1
  [Va] -> Fourier6/1
  Divide3/1 -> To Workspace2/1, Display2/1
  Fourier3/1 -> Magnitude-Angle to Complex3/1
  Degrees to Radians6/1 -> Magnitude-Angle to Complex6/2
  Divide2/1 -> [Za], To Workspace/1, Display/1
  Fourier6/1 -> Magnitude-Angle to Complex6/1
  Fourier8/1 -> Magnitude-Angle to Complex8/1
  Fourier2/2 -> Degrees to Radians2/1
  Fourier3/2 -> Degrees to Radians3/1
  Degrees to Radians1/1 -> Magnitude-Angle to Complex1/2
  [Vc] -> Fourier3/1
  Magnitude-Angle to Complex4/1 -> Divide3/2
  Fourier4/1 -> Magnitude-Angle to Complex4/1
  Fourier1/1 -> Magnitude-Angle to Complex1/1
  Degrees to Radians3/1 -> Magnitude-Angle to Complex3/2
  [Ic] -> Fourier4/1
  Magnitude-Angle to Complex2/1 -> Divide1/2
  Magnitude-Angle to Complex1/1 -> Divide1/1
  Fourier1/2 -> Degrees to Radians1/1
  [Vb] -> Fourier1/1
  Fourier2/1 -> Magnitude-Angle to Complex2/1

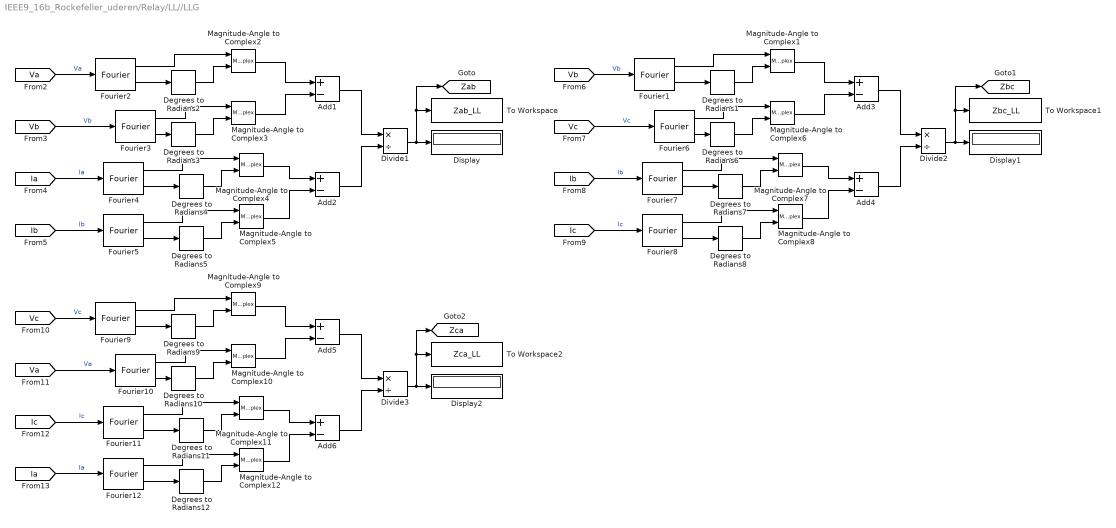
== system IEEE9_16b_Rockefeller_uderen/Relay/LL//LLG ==
  Add{1..6} (6 alike) : Sum  Inputs=+-
  Degrees to Radians{1..12} (12 alike) : simulink_extras/Transformations/Degrees to Radians
  Display : Display
  Display1 : Display
  Display2 : Display
  Divide1 : Product  Inputs=*/
  Divide2 : Product  Inputs=*/
  Divide3 : Product  Inputs=*/
  Fourier{1..12} (12 alike) : powerlib_meascontrol/Measurements/Fourier  Freq=60  n=1  InInit=[0, 0]  Ts=0
  Magnitude-Angle to Complex{1..12} (12 alike) : MagnitudeAngleToComplex
  To Workspace : ToWorkspace  VariableName=Zab_LL  SaveFormat=Timeseries  SampleTime=-1
  To Workspace1 : ToWorkspace  VariableName=Zbc_LL  SaveFormat=Timeseries  SampleTime=-1
  To Workspace2 : ToWorkspace  VariableName=Zca_LL  SaveFormat=Timeseries  SampleTime=-1
  tag scope: Zab=global, Zbc=global, Zca=global
  wires:
  Fourier12/2 -> Degrees to Radians12/1
  [Vc] -> Fourier9/1  "Vc"
  [Vc] -> Fourier6/1  "Vc"
  Magnitude-Angle to Complex11/1 -> Add6/1
  Fourier2/2 -> Degrees to Radians2/1
  Degrees to Radians8/1 -> Magnitude-Angle to Complex8/2
  Fourier10/1 -> Magnitude-Angle to Complex10/1
  Magnitude-Angle to Complex5/1 -> Add2/2
  Add1/1 -> Divide1/1
  Magnitude-Angle to Complex10/1 -> Add5/2
  Fourier3/2 -> Degrees to Radians3/1
  Degrees to Radians7/1 -> Magnitude-Angle to Complex7/2
  Divide2/1 -> Display1/1, [Zbc], To Workspace1/1
  [Va] -> Fourier2/1  "Va"
  Degrees to Radians6/1 -> Magnitude-Angle to Complex6/2
  [Vb] -> Fourier1/1  "Vb"
  Fourier1/2 -> Degrees to Radians1/1
  Fourier3/1 -> Magnitude-Angle to Complex3/1
  [Ib] -> Fourier7/1  "Ib"
  Divide1/1 -> [Zab], To Workspace/1, Display/1
  Degrees to Radians5/1 -> Magnitude-Angle to Complex5/2
  Magnitude-Angle to Complex2/1 -> Add1/1
  Degrees to Radians10/1 -> Magnitude-Angle to Complex10/2
  Fourier8/2 -> Degrees to Radians8/1
  Add3/1 -> Divide2/1
  Fourier8/1 -> Magnitude-Angle to Complex8/1
  [Ic] -> Fourier11/1  "Ic"
  Fourier6/2 -> Degrees to Radians6/1
  Fourier7/2 -> Degrees to Radians7/1
  Fourier5/1 -> Magnitude-Angle to Complex5/1
  [Ic] -> Fourier8/1  "Ic"
  Fourier10/2 -> Degrees to Radians10/1
  Fourier11/2 -> Degrees to Radians11/1
  Degrees to Radians2/1 -> Magnitude-Angle to Complex2/2
  Fourier11/1 -> Magnitude-Angle to Complex11/1
  [Ib] -> Fourier5/1  "Ib"
  Fourier6/1 -> Magnitude-Angle to Complex6/1
  Degrees to Radians3/1 -> Magnitude-Angle to Complex3/2
  Degrees to Radians11/1 -> Magnitude-Angle to Complex11/2
  Fourier7/1 -> Magnitude-Angle to Complex7/1
  Magnitude-Angle to Complex6/1 -> Add3/2
  Fourier2/1 -> Magnitude-Angle to Complex2/1
  Magnitude-Angle to Complex12/1 -> Add6/2
  Magnitude-Angle to Complex8/1 -> Add4/2
  Degrees to Radians9/1 -> Magnitude-Angle to Complex9/2
  [Vb] -> Fourier3/1  "Vb"
  Fourier4/1 -> Magnitude-Angle to Complex4/1
  Add4/1 -> Divide2/2
  Degrees to Radians1/1 -> Magnitude-Angle to Complex1/2
  [Va] -> Fourier10/1  "Va"
  Magnitude-Angle to Complex9/1 -> Add5/1
  Fourier1/1 -> Magnitude-Angle to Complex1/1
  Magnitude-Angle to Complex7/1 -> Add4/1
  [Ia] -> Fourier4/1  "Ia"
  Add2/1 -> Divide1/2
  [Ia] -> Fourier12/1  "Ia"
  Degrees to Radians4/1 -> Magnitude-Angle to Complex4/2
  Fourier4/2 -> Degrees to Radians4/1
  Magnitude-Angle to Complex3/1 -> Add1/2
  Fourier12/1 -> Magnitude-Angle to Complex12/1
  Add6/1 -> Divide3/2
  Degrees to Radians12/1 -> Magnitude-Angle to Complex12/2
  Magnitude-Angle to Complex1/1 -> Add3/1
  Fourier9/2 -> Degrees to Radians9/1
  Add5/1 -> Divide3/1
  Magnitude-Angle to Complex4/1 -> Add2/1
  Fourier5/2 -> Degrees to Radians5/1
  Fourier9/1 -> Magnitude-Angle to Complex9/1
  Divide3/1 -> [Zca], To Workspace2/1, Display2/1

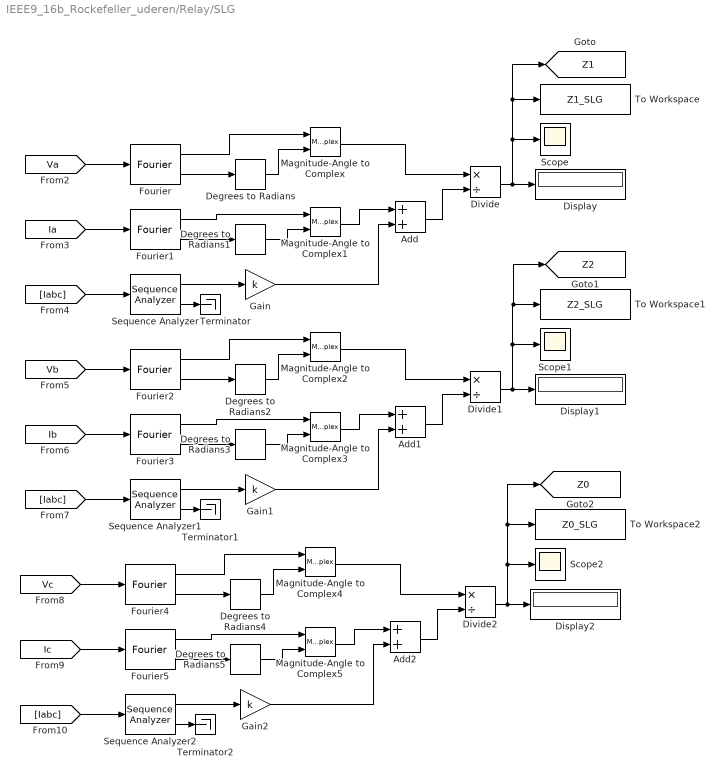
== system IEEE9_16b_Rockefeller_uderen/Relay/SLG ==
  Add : Sum
  Add1 : Sum
  Add2 : Sum
  Degrees to Radians{,1..5} (6 alike) : simulink_extras/Transformations/Degrees to Radians
  Display : Display
  Display1 : Display
  Display2 : Display
  Divide : Product  Inputs=*/
  Divide1 : Product  Inputs=*/
  Divide2 : Product  Inputs=*/
  Fourier{,1..5} (6 alike) : powerlib_meascontrol/Measurements/Fourier  Freq=60  n=1  InInit=[0, 0]  Ts=0
  Gain : Gain  Gain=k
  Gain1 : Gain  Gain=k
  Gain2 : Gain  Gain=k
  Magnitude-Angle to Complex{,1..5} (6 alike) : MagnitudeAngleToComplex
  Scope : Scope
  Scope1 : Scope
  Scope2 : Scope
  Sequence Analyzer : powerlib_meascontrol/Measurements/Sequence Analyzer  Freq=60  n=1  seq=Zero  InInit=[1, 0]  Ts=0
      settings: SourceProductBaseCode=PS
  Sequence Analyzer1 : powerlib_meascontrol/Measurements/Sequence Analyzer  Freq=60  n=1  seq=Zero  InInit=[1, 0]  Ts=0
      settings: SourceProductBaseCode=PS
  Sequence Analyzer2 : powerlib_meascontrol/Measurements/Sequence Analyzer  Freq=60  n=1  seq=Zero  InInit=[1, 0]  Ts=0
      settings: SourceProductBaseCode=PS
  Terminator : Terminator
  Terminator1 : Terminator
  Terminator2 : Terminator
  To Workspace : ToWorkspace  VariableName=Z1_SLG  SaveFormat=Timeseries  SampleTime=-1
  To Workspace1 : ToWorkspace  VariableName=Z2_SLG  SaveFormat=Timeseries  SampleTime=-1
  To Workspace2 : ToWorkspace  VariableName=Z0_SLG  SaveFormat=Timeseries  SampleTime=-1
  tag scope: Z0=global, Z1=global, Z2=global
  wires:
  Gain/1 -> Add/2
  Gain1/1 -> Add1/2
  Magnitude-Angle to Complex3/1 -> Add1/1
  Fourier1/2 -> Degrees to Radians1/1
  Sequence Analyzer1/1 -> Gain1/1
  [Va] -> Fourier/1
  Sequence Analyzer2/1 -> Gain2/1
  Magnitude-Angle to Complex/1 -> Divide/1
  Fourier1/1 -> Magnitude-Angle to Complex1/1
  Degrees to Radians/1 -> Magnitude-Angle to Complex/2
  Add/1 -> Divide/2
  Sequence Analyzer/1 -> Gain/1
  [Ib] -> Fourier3/1
  Fourier3/2 -> Degrees to Radians3/1
  Add1/1 -> Divide1/2
  Divide2/1 -> [Z0], To Workspace2/1, Scope2/1, Display2/1
  Fourier/1 -> Magnitude-Angle to Complex/1
  [Iabc] -> Sequence Analyzer/1
  Add2/1 -> Divide2/2
  Fourier4/2 -> Degrees to Radians4/1
  Magnitude-Angle to Complex1/1 -> Add/1
  Fourier/2 -> Degrees to Radians/1
  Degrees to Radians5/1 -> Magnitude-Angle to Complex5/2
  Degrees to Radians1/1 -> Magnitude-Angle to Complex1/2
  [Ia] -> Fourier1/1
  Divide1/1 -> Display1/1, Scope1/1, [Z2], To Workspace1/1
  Divide/1 -> [Z1], To Workspace/1, Scope/1, Display/1
  Degrees to Radians3/1 -> Magnitude-Angle to Complex3/2
  Magnitude-Angle to Complex2/1 -> Divide1/1
  Fourier4/1 -> Magnitude-Angle to Complex4/1
  [Vc] -> Fourier4/1
  Sequence Analyzer1/2 -> Terminator1/1
  Degrees to Radians2/1 -> Magnitude-Angle to Complex2/2
  Sequence Analyzer2/2 -> Terminator2/1
  Fourier3/1 -> Magnitude-Angle to Complex3/1
  Gain2/1 -> Add2/2
  [Ic] -> Fourier5/1
  Fourier2/1 -> Magnitude-Angle to Complex2/1
  Degrees to Radians4/1 -> Magnitude-Angle to Complex4/2
  Magnitude-Angle to Complex5/1 -> Add2/1
  [Iabc] -> Sequence Analyzer1/1
  [Vb] -> Fourier2/1
  Fourier2/2 -> Degrees to Radians2/1
  Sequence Analyzer/2 -> Terminator/1
  Fourier5/1 -> Magnitude-Angle to Complex5/1
  Fourier5/2 -> Degrees to Radians5/1
  Magnitude-Angle to Complex4/1 -> Divide2/1
  [Iabc] -> Sequence Analyzer2/1

== matlab function IEEE9_16b_Rockefeller_uderen/Relay/MATLAB Function ==
  settings: updateMethod=DISCRETE
  data: Vabc input; Za output; Iabc input; Zb output; Zc output; Zab output; Zbc output; Zca output; Za_3ph output; Zb_3ph output; Zc_3ph output; T1 output; T2 output; T3 output
function [Za, Zb, Zc, Zab, Zbc, Zca, Za_3ph, Zb_3ph, Zc_3ph, T1, T2, T3] = fcn(Vabc, Iabc)
 
persistent init C1 C2 C3 r1 r2 r3 trip1 trip2 trip3 k
if isempty(init)  
    trip1 = false; trip2 = false; trip3 = false;
    Zline = 100*(0.0449 + 1i*2*pi*60*1.01e-3);
    Z0_line = 100*(0.11241 + 1i*60*2.02e-3*2*pi);
    k = (Z0_line - Zline)./Zline;
    Z1 = 0.80*Zline;
    Z2 = 1.2*Zline;
    Z3 = 2*abs(Zline)*exp(1i*80*pi/180);
    C1 = Z1/2; C2 = Z2/2; C3 = Z3/2;
    r1 = abs(C1); r2 = abs(C2); r3 = abs(C3);
    MTA1 = angle(Z1);
    MTA2 = angle(Z2);
    MTA3 = 80*pi/180;
    init = 1;
    
%     circle(real(C1),imag(C1),r1)
%     circle(real(C2),imag(C2),r2)
%     circle(real(C3),imag(C3),r3)
end

Va = Vabc(1); Vb = Vabc(2); Vc = Vabc(3);
Ia = Iabc(1); Ib = Iabc(2); Ic =Iabc(3);
Io = (Ia+Ib+Ic)/3;

Za = Va/(Ia+k*Io);
Zb = Vb/(Ib+k*Io);
Zc = Vc/(Ic+k*Io);
Zab = (Va-Vb)/(Ia-Ib);
Zbc = (Vb-Vc)/(Ib-Ic);
Zca = (Vc-Va)/(Ic-Ia);
Za_3ph = Va/Ia;
Zb_3ph = Vb/Ib;
Zc_3ph = Vc/Ic;

if any([abs(Za-C1),abs(Zb-C1),abs(Zc-C1),abs(Zab-C1),abs(Zbc-C1),abs(Zca-C1),abs(Za_3ph-C1),abs(Zb_3ph-C1),abs(Zc_3ph-C1)] <= r1)
    trip1 = true;
elseif any([abs(Za-C2),abs(Zb-C2),abs(Zc-C2),abs(Zab-C2),abs(Zbc-C2),abs(Zca-C2),abs(Za_3ph-C2),abs(Zb_3ph-C2),abs(Zc_3ph-C2)] <= r2)
    trip2 = true;
elseif any([abs(Za-C3),abs(Zb-C3),abs(Zc-C3),abs(Zab-C3),abs(Zbc-C3),abs(Zca-C3),abs(Za_3ph-C3),abs(Zb_3ph-C3),abs(Zc_3ph-C3)] <= r3)
    trip3 = true;
end

T1 =trip1; T2 = trip2; T3 = trip3;
end
